simulink model "m"  (R2021b)
settings: Solver=VariableStepAuto  StartTime=0.0  StopTime=10.0  RelTol=1e-3
undefined symbols (not defined in the file): k1, k2, m1, m2, m3
settings Model: Creator=szczy  LastModifiedBy=szczy

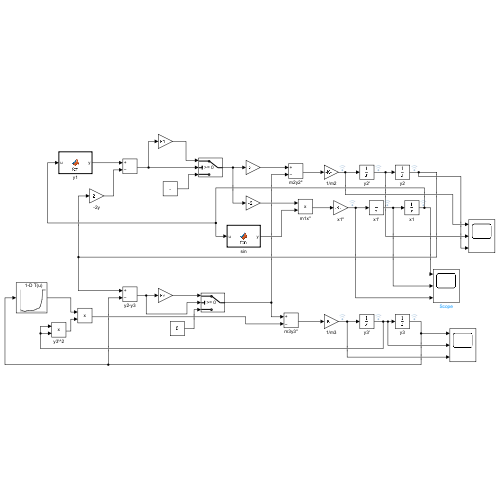
[thumbnail: Simulink's stored preview of the top-level diagram]
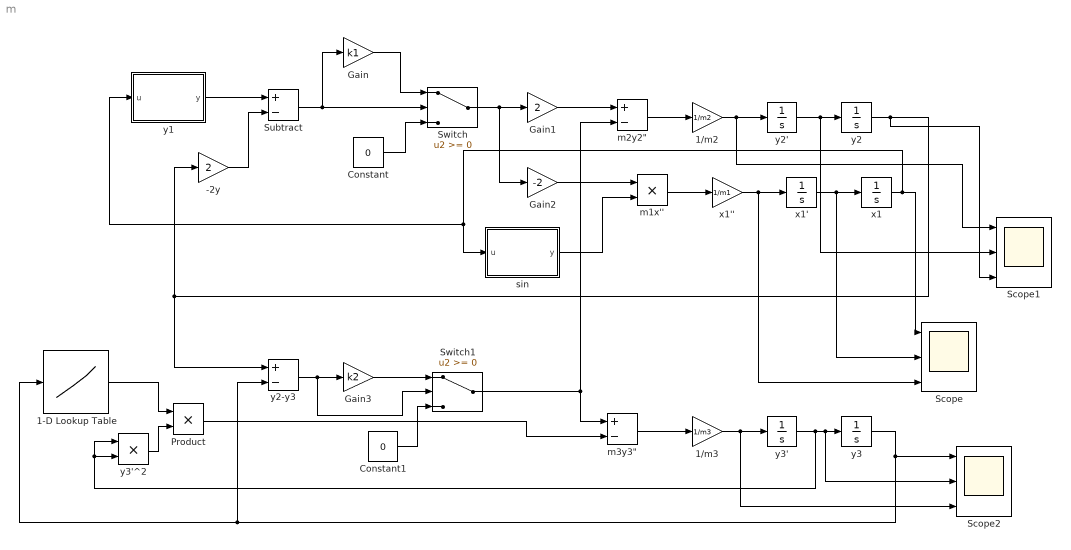
== system m ==
  -2y : Gain  Gain=2
  1-D Lookup Table : Lookup_n-D  NumberOfTableDimensions=1  BreakpointsForDimension1=[0, 10, 20, 30, 40, 50, 60, 70, 80, 90, 94, 98, 102, 104, 107, 120]  Table=[833, 400, 160, 320, 520, 520, 660, 830, 1070, 1600, 2100, 2800, 4100, 5000, 9000, 9000]  InternalRulePriority=Speed  RndMeth=Simplest  InputSameDT=on
  1/m2 : Gain  Gain=1/m2
  1/m3 : Gain  Gain=1/m3
  Constant : Constant  Value=0
  Constant1 : Constant  Value=0
  Gain : Gain  Gain=k1
  Gain1 : Gain  Gain=2
  Gain2 : Gain  Gain=-2
  Gain3 : Gain  Gain=k2
  Product : Product
  Scope : Scope  NumInputPorts=3
  Scope1 : Scope  NumInputPorts=3
  Scope2 : Scope  NumInputPorts=3
  Subtract : Sum  Inputs=+-
  Switch : Switch
  Switch1 : Switch
  m1x'' : Product
  "m2y2\"" : Sum  Inputs=+-
  "m3y3\"" : Sum  Inputs=+-
  sin : MATLAB Function  TreatAsAtomicUnit=on
  x1 : Integrator
  x1' : Integrator  InitialCondition=67
  x1'' : Gain  Gain=1/m1
  y1 : MATLAB Function  TreatAsAtomicUnit=on
  y2 : Integrator
  y2' : Integrator
  y2-y3 : Sum  Inputs=+-
  y3 : Integrator
  y3' : Integrator
  y3'^2 : Product
  wires:
  -2y/1 -> Subtract/2
  Constant/1 -> Switch/3
  Subtract/1 -> Gain/1, Switch/2
  Gain/1 -> Switch/1
  Switch/1 -> Gain2/1, Gain1/1
  Gain1/1 -> "m2y2\""/1
  Gain2/1 -> m1x''/1
  sin/1(y) -> m1x''/2
  m1x''/1 -> x1''/1
  x1''/1 -> Scope/3, x1'/1
  x1'/1 -> Scope/2, x1/1
  x1/1 -> Scope/1, y1/1(u), sin/1(u)
  1/m2/1 -> Scope1/1, y2'/1
  y2'/1 -> Scope1/2, y2/1
  "m2y2\""/1 -> 1/m2/1
  y2/1 -> Scope1/3, y2-y3/1, -2y/1
  y2-y3/1 -> Switch1/2, Gain3/1
  Gain3/1 -> Switch1/1
  Constant1/1 -> Switch1/3
  Switch1/1 -> "m3y3\""/1, "m2y2\""/2
  "m3y3\""/1 -> 1/m3/1
  y3'/1 -> y3'^2/1, y3'^2/2, Scope2/2, y3/1
  1/m3/1 -> Scope2/3, y3'/1
  y3'^2/1 -> Product/2
  1-D Lookup Table/1 -> Product/1
  Product/1 -> "m3y3\""/2
  y3/1 -> Scope2/1, 1-D Lookup Table/1, y2-y3/2
  y1/1(y) -> Subtract/1

== matlab function m/y1 ==
  data: u input; y output
function y = fcn(u)

y = sqrt(u^2 + 42^2) - 42;

== matlab function m/sin ==
  data: u input; y output
function y = fcn(u)

y = u / sqrt(u^2 + 42^2);
